simulink model "simulink_rcl_devre1"  (R2013a)
settings: Solver=ode45  StartTime=0.0  StopTime=10.0  RelTol=1e-3
settings Model: Creator=alper pc  LastModifiedBy=alper pc

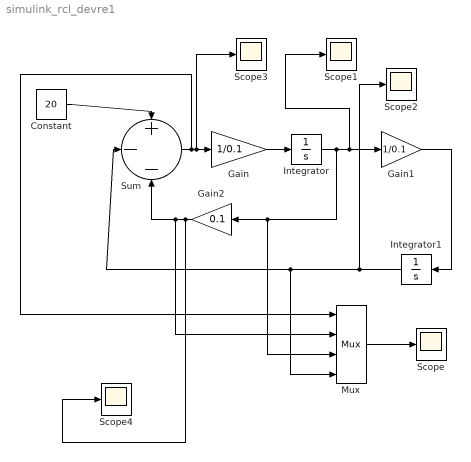
== system simulink_rcl_devre1 ==
  Constant : Constant  Value=20
  Gain : Gain  Gain=1/0.1
  Gain1 : Gain  Gain=1/0.1
  Gain2 : Gain  Gain=0.1
  Integrator : Integrator
  Integrator1 : Integrator
  Mux : Mux
  Scope{,1..4} (5 alike) : Scope
      Scope2 settings: SaveName=ScopeData2
      Scope3 settings: SaveName=ScopeData3
      Scope4 settings: SaveName=ScopeData4
  Sum : Sum  Inputs=+--
  wires:
  Constant/1 -> Sum/1
  Sum/1 -> Mux/1, Scope3/1, Gain/1
  Gain/1 -> Integrator/1
  Integrator/1 -> Mux/3, Gain2/1, Scope1/1, Gain1/1
  Gain1/1 -> Integrator1/1
  Integrator1/1 -> Scope2/1, Mux/4, Sum/2
  Gain2/1 -> Scope4/1, Mux/2, Sum/3
  Mux/1 -> Scope/1
